simulink library "Simple_lib"  (R2018b)
settings: Solver=ode45  StartTime=0.0  StopTime=10.0  RelTol=1e-3  EnableMultiTasking=on
undefined symbols (not defined in the file or in its folder): Acceptance, beta, C, C_J, C_P, c_wall, dGain, DiscIntNeverNeededParam, Duplex, Electrical_lib, grab, h_fe, i, i3, K_T, Kman, KmanCE, mu_s, n_rev, R_arm, Simplex, systemTs, tau_0, TinIC, Ts, w_0, wallMass, Watch_lib
libraries: $bdroot x407, PlantUtilityBlockset_lib x30, peGeneralControl x22, simulink x11
(part 10 of 14)

== system Simple_lib/Utility/SimplexSav ==
  InPot : Inport
  InFlow : Inport  Tag=NOFLUX  Port=2
  FlowDisplay : Display
  FlowSimplexPlexGraphix2 : Scope
      settings: Tag=Flow
  PotDisplay : Display
  PotSimplexPlexGraphix2 : Scope
      settings: Tag=Pot
  Rate Transition : RateTransition  OutPortSampleTimeMultiple=Ts  OutPortSampleTime=Ts
  OutPot : Outport  Tag=NOFLUX
  tag scope: SimplexSubsystemPlexGraphix2=global
  wires:
  InPot/1 -> Rate Transition/1
  InFlow/1 -> FlowSimplexPlexGraphix2/1, FlowDisplay/1, [SimplexSubsystemPlexGraphix2]
  Rate Transition/1 -> OutPot/1, PotSimplexPlexGraphix2/1, PotDisplay/1

== system Simple_lib/Driveline/Changan Transmission/EMachine ==
  J_eMotor : Subsystem  AncestorBlock=PlantUtilityBlockset_lib/Driveline/InertialState
      mask Display:
      | %color('white');
      | %plot([-1 4],[1 1]);
      | %plot([-1 4],[-1 -1]);
      | %color('black')
      | %plot([1 4],[0 0]);
      | plot([-1 -.9 -.5 0 .5 .9 1  .9  .5  0 -.5 -.9 -1],      [ 0  .5 .9 1 .9 .5 0 -.5 -.9 -1 -.9 -.5  0]);
      | %plot([4 4.5 4.5 4],[0 -0.25 0.25 0])
  Transducer : Subsystem
  V : Outport
  w : Outport  Port=2
  wires:
  J_eMotor/1(Out1) -> w/1, Transducer/1(w)
  Transducer/1(V) -> V/1

== system Simple_lib/Driveline/Changan Transmission/FD1 ==
  In1 : Inport
  Pull : Subsystem  Tag=Electrical  AncestorBlock=PlantUtilityBlockset_lib/Utility/Pull  InitFcn=initDuplex
      mask Display:
      | color('white')
      | plot([0 3], [2 2])
      | plot([0 3], [-2 -2])
      | color('black')
      | 
      | plot([0 1 1], [0 0 0.4])
      | plot([1 1 3], [0.6 1 1])
      | plot([1 3 2 1 0 2], [0.6 0.6 0.4 0.6 0.4 0.4])
      | patch([0 2 1],[0.4 0.4 0.6],[0,0,0])
      | plot([3 2 2], [1 1 0.6])
      | plot([2 2 3], [0.4 -1 -1])
  Push : Subsystem  AncestorBlock=PlantUtilityBlockset_lib/Utility/Push  InitFcn=initSimplex
      mask Display:
      | color('white')
      | plot([0 3], [2 2])
      | plot([0 3], [-2 -2])
      | color('black')
      | 
      | plot([0 2 2 3], [1 1 0 0])
      | plot([1 3 2 1 0 2], [0.6 0.6 0.4 0.6 0.4 0.4])
      | patch([1 3 2],[0.6 0.6 0.4],[0,0,0])
      | plot([0 1 1], [1 1 0.6])
      | plot([1 1 0], [0.4 -1 -1])
  ratio : Gain  Gain=n_i/n_o
  speed ratio : Gain  Gain=n_i/n_o
  Out1 : Outport
  wires:
  Pull/1(OutPot) -> Out1/1
  In1/1 -> Push/1(InPot)
  ratio/1 -> Push/2(InFlow)
  Pull/2(OutFlow) -> ratio/1
  speed ratio/1 -> Pull/1(InPot)
  Push/1(OutPot) -> speed ratio/1

== system Simple_lib/Driveline/Changan Transmission/FD2 ==
  In1 : Inport
  Pull : Subsystem  Tag=Electrical  AncestorBlock=PlantUtilityBlockset_lib/Utility/Pull  InitFcn=initDuplex
      mask Display:
      | color('white')
      | plot([0 3], [2 2])
      | plot([0 3], [-2 -2])
      | color('black')
      | 
      | plot([0 1 1], [0 0 0.4])
      | plot([1 1 3], [0.6 1 1])
      | plot([1 3 2 1 0 2], [0.6 0.6 0.4 0.6 0.4 0.4])
      | patch([0 2 1],[0.4 0.4 0.6],[0,0,0])
      | plot([3 2 2], [1 1 0.6])
      | plot([2 2 3], [0.4 -1 -1])
  Push : Subsystem  AncestorBlock=PlantUtilityBlockset_lib/Utility/Push  InitFcn=initSimplex
      mask Display:
      | color('white')
      | plot([0 3], [2 2])
      | plot([0 3], [-2 -2])
      | color('black')
      | 
      | plot([0 2 2 3], [1 1 0 0])
      | plot([1 3 2 1 0 2], [0.6 0.6 0.4 0.6 0.4 0.4])
      | patch([1 3 2],[0.6 0.6 0.4],[0,0,0])
      | plot([0 1 1], [1 1 0.6])
      | plot([1 1 0], [0.4 -1 -1])
  ratio : Gain  Gain=n_i/n_o
  speed ratio : Gain  Gain=n_i/n_o
  Out1 : Outport
  wires:
  Pull/1(OutPot) -> Out1/1
  In1/1 -> Push/1(InPot)
  ratio/1 -> Push/2(InFlow)
  Pull/2(OutFlow) -> ratio/1
  speed ratio/1 -> Pull/1(InPot)
  Push/1(OutPot) -> speed ratio/1

== system Simple_lib/Driveline/Changan Transmission/GP1 ==
  In1 : Inport
  Pull : Subsystem  Tag=Electrical  AncestorBlock=PlantUtilityBlockset_lib/Utility/Pull  InitFcn=initDuplex
      mask Display:
      | color('white')
      | plot([0 3], [2 2])
      | plot([0 3], [-2 -2])
      | color('black')
      | 
      | plot([0 1 1], [0 0 0.4])
      | plot([1 1 3], [0.6 1 1])
      | plot([1 3 2 1 0 2], [0.6 0.6 0.4 0.6 0.4 0.4])
      | patch([0 2 1],[0.4 0.4 0.6],[0,0,0])
      | plot([3 2 2], [1 1 0.6])
      | plot([2 2 3], [0.4 -1 -1])
  Push : Subsystem  AncestorBlock=PlantUtilityBlockset_lib/Utility/Push  InitFcn=initSimplex
      mask Display:
      | color('white')
      | plot([0 3], [2 2])
      | plot([0 3], [-2 -2])
      | color('black')
      | 
      | plot([0 2 2 3], [1 1 0 0])
      | plot([1 3 2 1 0 2], [0.6 0.6 0.4 0.6 0.4 0.4])
      | patch([1 3 2],[0.6 0.6 0.4],[0,0,0])
      | plot([0 1 1], [1 1 0.6])
      | plot([1 1 0], [0.4 -1 -1])
  ratio : Gain  Gain=n_i/n_o
  speed ratio : Gain  Gain=n_i/n_o
  Out1 : Outport
  wires:
  Pull/1(OutPot) -> Out1/1
  In1/1 -> Push/1(InPot)
  ratio/1 -> Push/2(InFlow)
  Pull/2(OutFlow) -> ratio/1
  speed ratio/1 -> Pull/1(InPot)
  Push/1(OutPot) -> speed ratio/1

== system Simple_lib/Driveline/Changan Transmission/GP2 ==
  In1 : Inport
  Pull : Subsystem  Tag=Electrical  AncestorBlock=PlantUtilityBlockset_lib/Utility/Pull  InitFcn=initDuplex
      mask Display:
      | color('white')
      | plot([0 3], [2 2])
      | plot([0 3], [-2 -2])
      | color('black')
      | 
      | plot([0 1 1], [0 0 0.4])
      | plot([1 1 3], [0.6 1 1])
      | plot([1 3 2 1 0 2], [0.6 0.6 0.4 0.6 0.4 0.4])
      | patch([0 2 1],[0.4 0.4 0.6],[0,0,0])
      | plot([3 2 2], [1 1 0.6])
      | plot([2 2 3], [0.4 -1 -1])
  Push : Subsystem  AncestorBlock=PlantUtilityBlockset_lib/Utility/Push  InitFcn=initSimplex
      mask Display:
      | color('white')
      | plot([0 3], [2 2])
      | plot([0 3], [-2 -2])
      | color('black')
      | 
      | plot([0 2 2 3], [1 1 0 0])
      | plot([1 3 2 1 0 2], [0.6 0.6 0.4 0.6 0.4 0.4])
      | patch([1 3 2],[0.6 0.6 0.4],[0,0,0])
      | plot([0 1 1], [1 1 0.6])
      | plot([1 1 0], [0.4 -1 -1])
  ratio : Gain  Gain=n_i/n_o
  speed ratio : Gain  Gain=n_i/n_o
  Out1 : Outport
  wires:
  Pull/1(OutPot) -> Out1/1
  In1/1 -> Push/1(InPot)
  ratio/1 -> Push/2(InFlow)
  Pull/2(OutFlow) -> ratio/1
  speed ratio/1 -> Pull/1(InPot)
  Push/1(OutPot) -> speed ratio/1

== system Simple_lib/Driveline/Changan Transmission/GP3 ==
  In1 : Inport
  Pull : Subsystem  Tag=Electrical  AncestorBlock=PlantUtilityBlockset_lib/Utility/Pull  InitFcn=initDuplex
      mask Display:
      | color('white')
      | plot([0 3], [2 2])
      | plot([0 3], [-2 -2])
      | color('black')
      | 
      | plot([0 1 1], [0 0 0.4])
      | plot([1 1 3], [0.6 1 1])
      | plot([1 3 2 1 0 2], [0.6 0.6 0.4 0.6 0.4 0.4])
      | patch([0 2 1],[0.4 0.4 0.6],[0,0,0])
      | plot([3 2 2], [1 1 0.6])
      | plot([2 2 3], [0.4 -1 -1])
  Push : Subsystem  AncestorBlock=PlantUtilityBlockset_lib/Utility/Push  InitFcn=initSimplex
      mask Display:
      | color('white')
      | plot([0 3], [2 2])
      | plot([0 3], [-2 -2])
      | color('black')
      | 
      | plot([0 2 2 3], [1 1 0 0])
      | plot([1 3 2 1 0 2], [0.6 0.6 0.4 0.6 0.4 0.4])
      | patch([1 3 2],[0.6 0.6 0.4],[0,0,0])
      | plot([0 1 1], [1 1 0.6])
      | plot([1 1 0], [0.4 -1 -1])
  ratio : Gain  Gain=n_i/n_o
  speed ratio : Gain  Gain=n_i/n_o
  Out1 : Outport
  wires:
  Pull/1(OutPot) -> Out1/1
  In1/1 -> Push/1(InPot)
  ratio/1 -> Push/2(InFlow)
  Pull/2(OutFlow) -> ratio/1
  speed ratio/1 -> Pull/1(InPot)
  Push/1(OutPot) -> speed ratio/1

== system Simple_lib/Driveline/Changan Transmission/GP4  ==
  In1 : Inport
  Pull : Subsystem  Tag=Electrical  AncestorBlock=PlantUtilityBlockset_lib/Utility/Pull  InitFcn=initDuplex
      mask Display:
      | color('white')
      | plot([0 3], [2 2])
      | plot([0 3], [-2 -2])
      | color('black')
      | 
      | plot([0 1 1], [0 0 0.4])
      | plot([1 1 3], [0.6 1 1])
      | plot([1 3 2 1 0 2], [0.6 0.6 0.4 0.6 0.4 0.4])
      | patch([0 2 1],[0.4 0.4 0.6],[0,0,0])
      | plot([3 2 2], [1 1 0.6])
      | plot([2 2 3], [0.4 -1 -1])
  Push : Subsystem  AncestorBlock=PlantUtilityBlockset_lib/Utility/Push  InitFcn=initSimplex
      mask Display:
      | color('white')
      | plot([0 3], [2 2])
      | plot([0 3], [-2 -2])
      | color('black')
      | 
      | plot([0 2 2 3], [1 1 0 0])
      | plot([1 3 2 1 0 2], [0.6 0.6 0.4 0.6 0.4 0.4])
      | patch([1 3 2],[0.6 0.6 0.4],[0,0,0])
      | plot([0 1 1], [1 1 0.6])
      | plot([1 1 0], [0.4 -1 -1])
  ratio : Gain  Gain=n_i/n_o
  speed ratio : Gain  Gain=n_i/n_o
  Out1 : Outport
  wires:
  Pull/1(OutPot) -> Out1/1
  In1/1 -> Push/1(InPot)
  ratio/1 -> Push/2(InFlow)
  Pull/2(OutFlow) -> ratio/1
  speed ratio/1 -> Pull/1(InPot)
  Push/1(OutPot) -> speed ratio/1

== system Simple_lib/Driveline/Changan Transmission/GP5 ==
  In1 : Inport
  Pull : Subsystem  Tag=Electrical  AncestorBlock=PlantUtilityBlockset_lib/Utility/Pull  InitFcn=initDuplex
      mask Display:
      | color('white')
      | plot([0 3], [2 2])
      | plot([0 3], [-2 -2])
      | color('black')
      | 
      | plot([0 1 1], [0 0 0.4])
      | plot([1 1 3], [0.6 1 1])
      | plot([1 3 2 1 0 2], [0.6 0.6 0.4 0.6 0.4 0.4])
      | patch([0 2 1],[0.4 0.4 0.6],[0,0,0])
      | plot([3 2 2], [1 1 0.6])
      | plot([2 2 3], [0.4 -1 -1])
  Push : Subsystem  AncestorBlock=PlantUtilityBlockset_lib/Utility/Push  InitFcn=initSimplex
      mask Display:
      | color('white')
      | plot([0 3], [2 2])
      | plot([0 3], [-2 -2])
      | color('black')
      | 
      | plot([0 2 2 3], [1 1 0 0])
      | plot([1 3 2 1 0 2], [0.6 0.6 0.4 0.6 0.4 0.4])
      | patch([1 3 2],[0.6 0.6 0.4],[0,0,0])
      | plot([0 1 1], [1 1 0.6])
      | plot([1 1 0], [0.4 -1 -1])
  ratio : Gain  Gain=n_i/n_o
  speed ratio : Gain  Gain=n_i/n_o
  Out1 : Outport
  wires:
  Pull/1(OutPot) -> Out1/1
  In1/1 -> Push/1(InPot)
  ratio/1 -> Push/2(InFlow)
  Pull/2(OutFlow) -> ratio/1
  speed ratio/1 -> Pull/1(InPot)
  Push/1(OutPot) -> speed ratio/1

== system Simple_lib/Driveline/Changan Transmission/GP6 ==
  In1 : Inport
  Pull : Subsystem  Tag=Electrical  AncestorBlock=PlantUtilityBlockset_lib/Utility/Pull  InitFcn=initDuplex
      mask Display:
      | color('white')
      | plot([0 3], [2 2])
      | plot([0 3], [-2 -2])
      | color('black')
      | 
      | plot([0 1 1], [0 0 0.4])
      | plot([1 1 3], [0.6 1 1])
      | plot([1 3 2 1 0 2], [0.6 0.6 0.4 0.6 0.4 0.4])
      | patch([0 2 1],[0.4 0.4 0.6],[0,0,0])
      | plot([3 2 2], [1 1 0.6])
      | plot([2 2 3], [0.4 -1 -1])
  Push : Subsystem  AncestorBlock=PlantUtilityBlockset_lib/Utility/Push  InitFcn=initSimplex
      mask Display:
      | color('white')
      | plot([0 3], [2 2])
      | plot([0 3], [-2 -2])
      | color('black')
      | 
      | plot([0 2 2 3], [1 1 0 0])
      | plot([1 3 2 1 0 2], [0.6 0.6 0.4 0.6 0.4 0.4])
      | patch([1 3 2],[0.6 0.6 0.4],[0,0,0])
      | plot([0 1 1], [1 1 0.6])
      | plot([1 1 0], [0.4 -1 -1])
  ratio : Gain  Gain=n_i/n_o
  speed ratio : Gain  Gain=n_i/n_o
  Out1 : Outport
  wires:
  Pull/1(OutPot) -> Out1/1
  In1/1 -> Push/1(InPot)
  ratio/1 -> Push/2(InFlow)
  Pull/2(OutFlow) -> ratio/1
  speed ratio/1 -> Pull/1(InPot)
  Push/1(OutPot) -> speed ratio/1

== system Simple_lib/Driveline/Changan Transmission/GPR ==
  In1 : Inport
  Pull : Subsystem  Tag=Electrical  AncestorBlock=PlantUtilityBlockset_lib/Utility/Pull  InitFcn=initDuplex
      mask Display:
      | color('white')
      | plot([0 3], [2 2])
      | plot([0 3], [-2 -2])
      | color('black')
      | 
      | plot([0 1 1], [0 0 0.4])
      | plot([1 1 3], [0.6 1 1])
      | plot([1 3 2 1 0 2], [0.6 0.6 0.4 0.6 0.4 0.4])
      | patch([0 2 1],[0.4 0.4 0.6],[0,0,0])
      | plot([3 2 2], [1 1 0.6])
      | plot([2 2 3], [0.4 -1 -1])
  Push : Subsystem  AncestorBlock=PlantUtilityBlockset_lib/Utility/Push  InitFcn=initSimplex
      mask Display:
      | color('white')
      | plot([0 3], [2 2])
      | plot([0 3], [-2 -2])
      | color('black')
      | 
      | plot([0 2 2 3], [1 1 0 0])
      | plot([1 3 2 1 0 2], [0.6 0.6 0.4 0.6 0.4 0.4])
      | patch([1 3 2],[0.6 0.6 0.4],[0,0,0])
      | plot([0 1 1], [1 1 0.6])
      | plot([1 1 0], [0.4 -1 -1])
  ratio : Gain  Gain=n_i/n_o
  speed ratio : Gain  Gain=n_i/n_o
  Out1 : Outport
  wires:
  Pull/1(OutPot) -> Out1/1
  In1/1 -> Push/1(InPot)
  ratio/1 -> Push/2(InFlow)
  Pull/2(OutFlow) -> ratio/1
  speed ratio/1 -> Pull/1(InPot)
  Push/1(OutPot) -> speed ratio/1

== system Simple_lib/Driveline/Changan Transmission/K0 ==
  w_in : Inport
  cap : Inport  Port=2
  w_out : Inport  Port=3
  1/R1 : Gain  Gain=-1
  1/R4 : Gain  Gain=-1
  Delay : Delay  DelayLength=1  InitialCondition=0
  Dw : Scope
  Dynamic Friction : Subsystem
  Push_in : Subsystem  AncestorBlock=PlantUtilityBlockset_lib/Utility/Push  InitFcn=initSimplex
      mask Display:
      | color('white')
      | plot([0 3], [2 2])
      | plot([0 3], [-2 -2])
      | color('black')
      | 
      | plot([0 2 2 3], [1 1 0 0])
      | plot([1 3 2 1 0 2], [0.6 0.6 0.4 0.6 0.4 0.4])
      | patch([1 3 2],[0.6 0.6 0.4],[0,0,0])
      | plot([0 1 1], [1 1 0.6])
      | plot([1 1 0], [0.4 -1 -1])
  Push_out : Subsystem  AncestorBlock=PlantUtilityBlockset_lib/Utility/Push  InitFcn=initSimplex
      mask Display:
      | color('white')
      | plot([0 3], [2 2])
      | plot([0 3], [-2 -2])
      | color('black')
      | 
      | plot([0 2 2 3], [1 1 0 0])
      | plot([1 3 2 1 0 2], [0.6 0.6 0.4 0.6 0.4 0.4])
      | patch([1 3 2],[0.6 0.6 0.4],[0,0,0])
      | plot([0 1 1], [1 1 0.6])
      | plot([1 1 0], [0.4 -1 -1])
  Static Friction : Subsystem
  Sum : Sum  Inputs=+|+
  Sum1 : Sum  Inputs=+|+
  Tq_Dyn : Scope
  Tq_stat : Scope
  Tq_trans : Scope
  capacity : Scope
  wires:
  w_out/1 -> Push_out/1(InPot)
  w_in/1 -> Push_in/1(InPot)
  1/R4/1 -> Sum/1
  Sum1/1 -> 1/R1/1, Delay/1, Push_in/2(InFlow)
  Sum/1 -> Dynamic Friction/1(Dw), Dw/1, Static Friction/2(Dw)
  Push_out/1(OutPot) -> Static Friction/3(w), Sum/2
  Push_in/1(OutPot) -> 1/R4/1
  Dynamic Friction/1(Tq_dyn) -> Tq_Dyn/1, Sum1/1
  Static Friction/1(Tq_stat) -> Tq_stat/1, Sum1/2
  Delay/1 -> Tq_trans/1, Static Friction/4(Tq)
  cap/1 -> capacity/1, Dynamic Friction/2(cap), Static Friction/1(cap)
  1/R1/1 -> Push_out/2(InFlow)

== system Simple_lib/Driveline/Changan Transmission/K1 ==
  w_in : Inport
  cap : Inport  Port=2
  w_out : Inport  Port=3
  1/R1 : Gain  Gain=-1
  1/R4 : Gain  Gain=-1
  Delay : Delay  DelayLength=1  InitialCondition=0
  Dw : Scope
  Dynamic Friction : Subsystem
  Push_in : Subsystem  AncestorBlock=PlantUtilityBlockset_lib/Utility/Push  InitFcn=initSimplex
      mask Display:
      | color('white')
      | plot([0 3], [2 2])
      | plot([0 3], [-2 -2])
      | color('black')
      | 
      | plot([0 2 2 3], [1 1 0 0])
      | plot([1 3 2 1 0 2], [0.6 0.6 0.4 0.6 0.4 0.4])
      | patch([1 3 2],[0.6 0.6 0.4],[0,0,0])
      | plot([0 1 1], [1 1 0.6])
      | plot([1 1 0], [0.4 -1 -1])
  Push_out : Subsystem  AncestorBlock=PlantUtilityBlockset_lib/Utility/Push  InitFcn=initSimplex
      mask Display:
      | color('white')
      | plot([0 3], [2 2])
      | plot([0 3], [-2 -2])
      | color('black')
      | 
      | plot([0 2 2 3], [1 1 0 0])
      | plot([1 3 2 1 0 2], [0.6 0.6 0.4 0.6 0.4 0.4])
      | patch([1 3 2],[0.6 0.6 0.4],[0,0,0])
      | plot([0 1 1], [1 1 0.6])
      | plot([1 1 0], [0.4 -1 -1])
  Static Friction : Subsystem
  Sum : Sum  Inputs=+|+
  Sum1 : Sum  Inputs=+|+
  Tq_Dyn : Scope
  Tq_stat : Scope
  Tq_trans : Scope
  capacity : Scope
  wires:
  w_out/1 -> Push_out/1(InPot)
  w_in/1 -> Push_in/1(InPot)
  1/R4/1 -> Sum/1
  Sum1/1 -> 1/R1/1, Delay/1, Push_in/2(InFlow)
  Sum/1 -> Dynamic Friction/1(Dw), Dw/1, Static Friction/2(Dw)
  Push_out/1(OutPot) -> Static Friction/3(w), Sum/2
  Push_in/1(OutPot) -> 1/R4/1
  Dynamic Friction/1(Tq_dyn) -> Tq_Dyn/1, Sum1/1
  Static Friction/1(Tq_stat) -> Tq_stat/1, Sum1/2
  Delay/1 -> Tq_trans/1, Static Friction/4(Tq)
  cap/1 -> capacity/1, Dynamic Friction/2(cap), Static Friction/1(cap)
  1/R1/1 -> Push_out/2(InFlow)

== system Simple_lib/Driveline/Changan Transmission/K2 ==
  w_in : Inport
  cap : Inport  Port=2
  w_out : Inport  Port=3
  1/R1 : Gain  Gain=-1
  1/R4 : Gain  Gain=-1
  Delay : Delay  DelayLength=1  InitialCondition=0
  Dw : Scope
  Dynamic Friction : Subsystem
  Push_in : Subsystem  AncestorBlock=PlantUtilityBlockset_lib/Utility/Push  InitFcn=initSimplex
      mask Display:
      | color('white')
      | plot([0 3], [2 2])
      | plot([0 3], [-2 -2])
      | color('black')
      | 
      | plot([0 2 2 3], [1 1 0 0])
      | plot([1 3 2 1 0 2], [0.6 0.6 0.4 0.6 0.4 0.4])
      | patch([1 3 2],[0.6 0.6 0.4],[0,0,0])
      | plot([0 1 1], [1 1 0.6])
      | plot([1 1 0], [0.4 -1 -1])
  Push_out : Subsystem  AncestorBlock=PlantUtilityBlockset_lib/Utility/Push  InitFcn=initSimplex
      mask Display:
      | color('white')
      | plot([0 3], [2 2])
      | plot([0 3], [-2 -2])
      | color('black')
      | 
      | plot([0 2 2 3], [1 1 0 0])
      | plot([1 3 2 1 0 2], [0.6 0.6 0.4 0.6 0.4 0.4])
      | patch([1 3 2],[0.6 0.6 0.4],[0,0,0])
      | plot([0 1 1], [1 1 0.6])
      | plot([1 1 0], [0.4 -1 -1])
  Static Friction : Subsystem
  Sum : Sum  Inputs=+|+
  Sum1 : Sum  Inputs=+|+
  Tq_Dyn : Scope
  Tq_stat : Scope
  Tq_trans : Scope
  capacity : Scope
  wires:
  w_out/1 -> Push_out/1(InPot)
  w_in/1 -> Push_in/1(InPot)
  1/R4/1 -> Sum/1
  Sum1/1 -> 1/R1/1, Delay/1, Push_in/2(InFlow)
  Sum/1 -> Dynamic Friction/1(Dw), Dw/1, Static Friction/2(Dw)
  Push_out/1(OutPot) -> Static Friction/3(w), Sum/2
  Push_in/1(OutPot) -> 1/R4/1
  Dynamic Friction/1(Tq_dyn) -> Tq_Dyn/1, Sum1/1
  Static Friction/1(Tq_stat) -> Tq_stat/1, Sum1/2
  Delay/1 -> Tq_trans/1, Static Friction/4(Tq)
  cap/1 -> capacity/1, Dynamic Friction/2(cap), Static Friction/1(cap)
  1/R1/1 -> Push_out/2(InFlow)

== system Simple_lib/Driveline/Changan Transmission/LoadScopes ==
  In1 : Inport
  Pull : Subsystem  Tag=Electrical  AncestorBlock=PlantUtilityBlockset_lib/Utility/Pull  InitFcn=initDuplex
      mask Display:
      | color('white')
      | plot([0 3], [2 2])
      | plot([0 3], [-2 -2])
      | color('black')
      | 
      | plot([0 1 1], [0 0 0.4])
      | plot([1 1 3], [0.6 1 1])
      | plot([1 3 2 1 0 2], [0.6 0.6 0.4 0.6 0.4 0.4])
      | patch([0 2 1],[0.4 0.4 0.6],[0,0,0])
      | plot([3 2 2], [1 1 0.6])
      | plot([2 2 3], [0.4 -1 -1])
  Push : Subsystem  AncestorBlock=PlantUtilityBlockset_lib/Utility/Push  InitFcn=initSimplex
      mask Display:
      | color('white')
      | plot([0 3], [2 2])
      | plot([0 3], [-2 -2])
      | color('black')
      | 
      | plot([0 2 2 3], [1 1 0 0])
      | plot([1 3 2 1 0 2], [0.6 0.6 0.4 0.6 0.4 0.4])
      | patch([1 3 2],[0.6 0.6 0.4],[0,0,0])
      | plot([0 1 1], [1 1 0.6])
      | plot([1 1 0], [0.4 -1 -1])
  Scope : Scope  NumInputPorts=2
  Out1 : Outport
  wires:
  Pull/1(OutPot) -> Out1/1
  In1/1 -> Push/1(InPot)
  Pull/2(OutFlow) -> Push/2(InFlow), Scope/2
  Push/1(OutPot) -> Scope/1, Pull/1(InPot)

== system Simple_lib/Driveline/Changan Transmission/Requirements ==
  note: Require synchroniser clutches to lock up when speeds across them are small for a while.
  note: Require clutches to lock up when speeds across them are small for a while.
  note: Require correct ratios when in each gear.
  In1 : Inport
  Out1 : Outport
  wires:
  In1/1 -> Out1/1

== system Simple_lib/Driveline/Changan Transmission/Shaft1 ==
  Discrete-Time Integrator1 : DiscreteIntegrator  gainval=1/5  SampleTime=Ts  ICPrevOutput=DiscIntNeverNeededParam  ICPrevScaledInput=DiscIntNeverNeededParam
  Pull : Subsystem  Tag=Electrical  AncestorBlock=PlantUtilityBlockset_lib/Utility/Pull  InitFcn=initDuplex
      mask Display:
      | color('white')
      | plot([0 3], [2 2])
      | plot([0 3], [-2 -2])
      | color('black')
      | 
      | plot([0 1 1], [0 0 0.4])
      | plot([1 1 3], [0.6 1 1])
      | plot([1 3 2 1 0 2], [0.6 0.6 0.4 0.6 0.4 0.4])
      | patch([0 2 1],[0.4 0.4 0.6],[0,0,0])
      | plot([3 2 2], [1 1 0.6])
      | plot([2 2 3], [0.4 -1 -1])
  Out1 : Outport
  wires:
  Discrete-Time Integrator1/1 -> Pull/1(InPot)
  Pull/2(OutFlow) -> Discrete-Time Integrator1/1
  Pull/1(OutPot) -> Out1/1

== system Simple_lib/Driveline/Changan Transmission/Shaft2 ==
  Discrete-Time Integrator1 : DiscreteIntegrator  gainval=1/5  SampleTime=Ts  ICPrevOutput=DiscIntNeverNeededParam  ICPrevScaledInput=DiscIntNeverNeededParam
  Pull : Subsystem  Tag=Electrical  AncestorBlock=PlantUtilityBlockset_lib/Utility/Pull  InitFcn=initDuplex
      mask Display:
      | color('white')
      | plot([0 3], [2 2])
      | plot([0 3], [-2 -2])
      | color('black')
      | 
      | plot([0 1 1], [0 0 0.4])
      | plot([1 1 3], [0.6 1 1])
      | plot([1 3 2 1 0 2], [0.6 0.6 0.4 0.6 0.4 0.4])
      | patch([0 2 1],[0.4 0.4 0.6],[0,0,0])
      | plot([3 2 2], [1 1 0.6])
      | plot([2 2 3], [0.4 -1 -1])
  Out1 : Outport
  wires:
  Discrete-Time Integrator1/1 -> Pull/1(InPot)
  Pull/2(OutFlow) -> Discrete-Time Integrator1/1
  Pull/1(OutPot) -> Out1/1

== system Simple_lib/Driveline/Changan Transmission/Synchro ==
  w_in : Inport
  cap : Inport  Port=2
  w_out : Inport  Port=3
  1/R1 : Gain  Gain=-1
  1/R4 : Gain  Gain=-1
  Delay : Delay  DelayLength=1  InitialCondition=0
  Dw : Scope
  Dynamic Friction : Subsystem
  Push_in : Subsystem  AncestorBlock=PlantUtilityBlockset_lib/Utility/Push  InitFcn=initSimplex
      mask Display:
      | color('white')
      | plot([0 3], [2 2])
      | plot([0 3], [-2 -2])
      | color('black')
      | 
      | plot([0 2 2 3], [1 1 0 0])
      | plot([1 3 2 1 0 2], [0.6 0.6 0.4 0.6 0.4 0.4])
      | patch([1 3 2],[0.6 0.6 0.4],[0,0,0])
      | plot([0 1 1], [1 1 0.6])
      | plot([1 1 0], [0.4 -1 -1])
  Push_out : Subsystem  AncestorBlock=PlantUtilityBlockset_lib/Utility/Push  InitFcn=initSimplex
      mask Display:
      | color('white')
      | plot([0 3], [2 2])
      | plot([0 3], [-2 -2])
      | color('black')
      | 
      | plot([0 2 2 3], [1 1 0 0])
      | plot([1 3 2 1 0 2], [0.6 0.6 0.4 0.6 0.4 0.4])
      | patch([1 3 2],[0.6 0.6 0.4],[0,0,0])
      | plot([0 1 1], [1 1 0.6])
      | plot([1 1 0], [0.4 -1 -1])
  Static Friction : Subsystem
  Sum : Sum  Inputs=+|+
  Sum1 : Sum  Inputs=+|+
  Tq_Dyn : Scope
  Tq_stat : Scope
  Tq_trans : Scope
  capacity : Scope
  wires:
  w_out/1 -> Push_out/1(InPot)
  w_in/1 -> Push_in/1(InPot)
  1/R4/1 -> Sum/1
  Sum1/1 -> 1/R1/1, Delay/1, Push_in/2(InFlow)
  Sum/1 -> Dynamic Friction/1(Dw), Dw/1, Static Friction/2(Dw)
  Push_out/1(OutPot) -> Static Friction/3(w), Sum/2
  Push_in/1(OutPot) -> 1/R4/1
  Dynamic Friction/1(Tq_dyn) -> Tq_Dyn/1, Sum1/1
  Static Friction/1(Tq_stat) -> Tq_stat/1, Sum1/2
  Delay/1 -> Tq_trans/1, Static Friction/4(Tq)
  cap/1 -> capacity/1, Dynamic Friction/2(cap), Static Friction/1(cap)
  1/R1/1 -> Push_out/2(InFlow)

== system Simple_lib/Driveline/Changan Transmission/Synchro1 ==
  w_in : Inport
  cap : Inport  Port=2
  w_out : Inport  Port=3
  1/R1 : Gain  Gain=-1
  1/R4 : Gain  Gain=-1
  Delay : Delay  DelayLength=1  InitialCondition=0
  Dw : Scope
  Dynamic Friction : Subsystem
  Push_in : Subsystem  AncestorBlock=PlantUtilityBlockset_lib/Utility/Push  InitFcn=initSimplex
      mask Display:
      | color('white')
      | plot([0 3], [2 2])
      | plot([0 3], [-2 -2])
      | color('black')
      | 
      | plot([0 2 2 3], [1 1 0 0])
      | plot([1 3 2 1 0 2], [0.6 0.6 0.4 0.6 0.4 0.4])
      | patch([1 3 2],[0.6 0.6 0.4],[0,0,0])
      | plot([0 1 1], [1 1 0.6])
      | plot([1 1 0], [0.4 -1 -1])
  Push_out : Subsystem  AncestorBlock=PlantUtilityBlockset_lib/Utility/Push  InitFcn=initSimplex
      mask Display:
      | color('white')
      | plot([0 3], [2 2])
      | plot([0 3], [-2 -2])
      | color('black')
      | 
      | plot([0 2 2 3], [1 1 0 0])
      | plot([1 3 2 1 0 2], [0.6 0.6 0.4 0.6 0.4 0.4])
      | patch([1 3 2],[0.6 0.6 0.4],[0,0,0])
      | plot([0 1 1], [1 1 0.6])
      | plot([1 1 0], [0.4 -1 -1])
  Static Friction : Subsystem
  Sum : Sum  Inputs=+|+
  Sum1 : Sum  Inputs=+|+
  Tq_Dyn : Scope
  Tq_stat : Scope
  Tq_trans : Scope
  capacity : Scope
  wires:
  w_out/1 -> Push_out/1(InPot)
  w_in/1 -> Push_in/1(InPot)
  1/R4/1 -> Sum/1
  Sum1/1 -> 1/R1/1, Delay/1, Push_in/2(InFlow)
  Sum/1 -> Dynamic Friction/1(Dw), Dw/1, Static Friction/2(Dw)
  Push_out/1(OutPot) -> Static Friction/3(w), Sum/2
  Push_in/1(OutPot) -> 1/R4/1
  Dynamic Friction/1(Tq_dyn) -> Tq_Dyn/1, Sum1/1
  Static Friction/1(Tq_stat) -> Tq_stat/1, Sum1/2
  Delay/1 -> Tq_trans/1, Static Friction/4(Tq)
  cap/1 -> capacity/1, Dynamic Friction/2(cap), Static Friction/1(cap)
  1/R1/1 -> Push_out/2(InFlow)

== system Simple_lib/Driveline/Changan Transmission/Synchro2 ==
  w_in : Inport
  cap : Inport  Port=2
  w_out : Inport  Port=3
  1/R1 : Gain  Gain=-1
  1/R4 : Gain  Gain=-1
  Delay : Delay  DelayLength=1  InitialCondition=0
  Dw : Scope
  Dynamic Friction : Subsystem
  Push_in : Subsystem  AncestorBlock=PlantUtilityBlockset_lib/Utility/Push  InitFcn=initSimplex
      mask Display:
      | color('white')
      | plot([0 3], [2 2])
      | plot([0 3], [-2 -2])
      | color('black')
      | 
      | plot([0 2 2 3], [1 1 0 0])
      | plot([1 3 2 1 0 2], [0.6 0.6 0.4 0.6 0.4 0.4])
      | patch([1 3 2],[0.6 0.6 0.4],[0,0,0])
      | plot([0 1 1], [1 1 0.6])
      | plot([1 1 0], [0.4 -1 -1])
  Push_out : Subsystem  AncestorBlock=PlantUtilityBlockset_lib/Utility/Push  InitFcn=initSimplex
      mask Display:
      | color('white')
      | plot([0 3], [2 2])
      | plot([0 3], [-2 -2])
      | color('black')
      | 
      | plot([0 2 2 3], [1 1 0 0])
      | plot([1 3 2 1 0 2], [0.6 0.6 0.4 0.6 0.4 0.4])
      | patch([1 3 2],[0.6 0.6 0.4],[0,0,0])
      | plot([0 1 1], [1 1 0.6])
      | plot([1 1 0], [0.4 -1 -1])
  Static Friction : Subsystem
  Sum : Sum  Inputs=+|+
  Sum1 : Sum  Inputs=+|+
  Tq_Dyn : Scope
  Tq_stat : Scope
  Tq_trans : Scope
  capacity : Scope
  wires:
  w_out/1 -> Push_out/1(InPot)
  w_in/1 -> Push_in/1(InPot)
  1/R4/1 -> Sum/1
  Sum1/1 -> 1/R1/1, Delay/1, Push_in/2(InFlow)
  Sum/1 -> Dynamic Friction/1(Dw), Dw/1, Static Friction/2(Dw)
  Push_out/1(OutPot) -> Static Friction/3(w), Sum/2
  Push_in/1(OutPot) -> 1/R4/1
  Dynamic Friction/1(Tq_dyn) -> Tq_Dyn/1, Sum1/1
  Static Friction/1(Tq_stat) -> Tq_stat/1, Sum1/2
  Delay/1 -> Tq_trans/1, Static Friction/4(Tq)
  cap/1 -> capacity/1, Dynamic Friction/2(cap), Static Friction/1(cap)
  1/R1/1 -> Push_out/2(InFlow)

== system Simple_lib/Driveline/Changan Transmission/Synchro3 ==
  w_in : Inport
  cap : Inport  Port=2
  w_out : Inport  Port=3
  1/R1 : Gain  Gain=-1
  1/R4 : Gain  Gain=-1
  Delay : Delay  DelayLength=1  InitialCondition=0
  Dw : Scope
  Dynamic Friction : Subsystem
  Push_in : Subsystem  AncestorBlock=PlantUtilityBlockset_lib/Utility/Push  InitFcn=initSimplex
      mask Display:
      | color('white')
      | plot([0 3], [2 2])
      | plot([0 3], [-2 -2])
      | color('black')
      | 
      | plot([0 2 2 3], [1 1 0 0])
      | plot([1 3 2 1 0 2], [0.6 0.6 0.4 0.6 0.4 0.4])
      | patch([1 3 2],[0.6 0.6 0.4],[0,0,0])
      | plot([0 1 1], [1 1 0.6])
      | plot([1 1 0], [0.4 -1 -1])
  Push_out : Subsystem  AncestorBlock=PlantUtilityBlockset_lib/Utility/Push  InitFcn=initSimplex
      mask Display:
      | color('white')
      | plot([0 3], [2 2])
      | plot([0 3], [-2 -2])
      | color('black')
      | 
      | plot([0 2 2 3], [1 1 0 0])
      | plot([1 3 2 1 0 2], [0.6 0.6 0.4 0.6 0.4 0.4])
      | patch([1 3 2],[0.6 0.6 0.4],[0,0,0])
      | plot([0 1 1], [1 1 0.6])
      | plot([1 1 0], [0.4 -1 -1])
  Static Friction : Subsystem
  Sum : Sum  Inputs=+|+
  Sum1 : Sum  Inputs=+|+
  Tq_Dyn : Scope
  Tq_stat : Scope
  Tq_trans : Scope
  capacity : Scope
  wires:
  w_out/1 -> Push_out/1(InPot)
  w_in/1 -> Push_in/1(InPot)
  1/R4/1 -> Sum/1
  Sum1/1 -> 1/R1/1, Delay/1, Push_in/2(InFlow)
  Sum/1 -> Dynamic Friction/1(Dw), Dw/1, Static Friction/2(Dw)
  Push_out/1(OutPot) -> Static Friction/3(w), Sum/2
  Push_in/1(OutPot) -> 1/R4/1
  Dynamic Friction/1(Tq_dyn) -> Tq_Dyn/1, Sum1/1
  Static Friction/1(Tq_stat) -> Tq_stat/1, Sum1/2
  Delay/1 -> Tq_trans/1, Static Friction/4(Tq)
  cap/1 -> capacity/1, Dynamic Friction/2(cap), Static Friction/1(cap)
  1/R1/1 -> Push_out/2(InFlow)

== system Simple_lib/Driveline/Changan Transmission/Synchro4 ==
  w_in : Inport
  cap : Inport  Port=2
  w_out : Inport  Port=3
  1/R1 : Gain  Gain=-1
  1/R4 : Gain  Gain=-1
  Delay : Delay  DelayLength=1  InitialCondition=0
  Dw : Scope
  Dynamic Friction : Subsystem
  Push_in : Subsystem  AncestorBlock=PlantUtilityBlockset_lib/Utility/Push  InitFcn=initSimplex
      mask Display:
      | color('white')
      | plot([0 3], [2 2])
      | plot([0 3], [-2 -2])
      | color('black')
      | 
      | plot([0 2 2 3], [1 1 0 0])
      | plot([1 3 2 1 0 2], [0.6 0.6 0.4 0.6 0.4 0.4])
      | patch([1 3 2],[0.6 0.6 0.4],[0,0,0])
      | plot([0 1 1], [1 1 0.6])
      | plot([1 1 0], [0.4 -1 -1])
  Push_out : Subsystem  AncestorBlock=PlantUtilityBlockset_lib/Utility/Push  InitFcn=initSimplex
      mask Display:
      | color('white')
      | plot([0 3], [2 2])
      | plot([0 3], [-2 -2])
      | color('black')
      | 
      | plot([0 2 2 3], [1 1 0 0])
      | plot([1 3 2 1 0 2], [0.6 0.6 0.4 0.6 0.4 0.4])
      | patch([1 3 2],[0.6 0.6 0.4],[0,0,0])
      | plot([0 1 1], [1 1 0.6])
      | plot([1 1 0], [0.4 -1 -1])
  Static Friction : Subsystem
  Sum : Sum  Inputs=+|+
  Sum1 : Sum  Inputs=+|+
  Tq_Dyn : Scope
  Tq_stat : Scope
  Tq_trans : Scope
  capacity : Scope
  wires:
  w_out/1 -> Push_out/1(InPot)
  w_in/1 -> Push_in/1(InPot)
  1/R4/1 -> Sum/1
  Sum1/1 -> 1/R1/1, Delay/1, Push_in/2(InFlow)
  Sum/1 -> Dynamic Friction/1(Dw), Dw/1, Static Friction/2(Dw)
  Push_out/1(OutPot) -> Static Friction/3(w), Sum/2
  Push_in/1(OutPot) -> 1/R4/1
  Dynamic Friction/1(Tq_dyn) -> Tq_Dyn/1, Sum1/1
  Static Friction/1(Tq_stat) -> Tq_stat/1, Sum1/2
  Delay/1 -> Tq_trans/1, Static Friction/4(Tq)
  cap/1 -> capacity/1, Dynamic Friction/2(cap), Static Friction/1(cap)
  1/R1/1 -> Push_out/2(InFlow)

== system Simple_lib/Driveline/Changan Transmission/Synchro5 ==
  w_in : Inport
  cap : Inport  Port=2
  w_out : Inport  Port=3
  1/R1 : Gain  Gain=-1
  1/R4 : Gain  Gain=-1
  Delay : Delay  DelayLength=1  InitialCondition=0
  Dw : Scope
  Dynamic Friction : Subsystem
  Push_in : Subsystem  AncestorBlock=PlantUtilityBlockset_lib/Utility/Push  InitFcn=initSimplex
      mask Display:
      | color('white')
      | plot([0 3], [2 2])
      | plot([0 3], [-2 -2])
      | color('black')
      | 
      | plot([0 2 2 3], [1 1 0 0])
      | plot([1 3 2 1 0 2], [0.6 0.6 0.4 0.6 0.4 0.4])
      | patch([1 3 2],[0.6 0.6 0.4],[0,0,0])
      | plot([0 1 1], [1 1 0.6])
      | plot([1 1 0], [0.4 -1 -1])
  Push_out : Subsystem  AncestorBlock=PlantUtilityBlockset_lib/Utility/Push  InitFcn=initSimplex
      mask Display:
      | color('white')
      | plot([0 3], [2 2])
      | plot([0 3], [-2 -2])
      | color('black')
      | 
      | plot([0 2 2 3], [1 1 0 0])
      | plot([1 3 2 1 0 2], [0.6 0.6 0.4 0.6 0.4 0.4])
      | patch([1 3 2],[0.6 0.6 0.4],[0,0,0])
      | plot([0 1 1], [1 1 0.6])
      | plot([1 1 0], [0.4 -1 -1])
  Static Friction : Subsystem
  Sum : Sum  Inputs=+|+
  Sum1 : Sum  Inputs=+|+
  Tq_Dyn : Scope
  Tq_stat : Scope
  Tq_trans : Scope
  capacity : Scope
  wires:
  w_out/1 -> Push_out/1(InPot)
  w_in/1 -> Push_in/1(InPot)
  1/R4/1 -> Sum/1
  Sum1/1 -> 1/R1/1, Delay/1, Push_in/2(InFlow)
  Sum/1 -> Dynamic Friction/1(Dw), Dw/1, Static Friction/2(Dw)
  Push_out/1(OutPot) -> Static Friction/3(w), Sum/2
  Push_in/1(OutPot) -> 1/R4/1
  Dynamic Friction/1(Tq_dyn) -> Tq_Dyn/1, Sum1/1
  Static Friction/1(Tq_stat) -> Tq_stat/1, Sum1/2
  Delay/1 -> Tq_trans/1, Static Friction/4(Tq)
  cap/1 -> capacity/1, Dynamic Friction/2(cap), Static Friction/1(cap)
  1/R1/1 -> Push_out/2(InFlow)

== system Simple_lib/Driveline/Changan Transmission/Synchro6 ==
  w_in : Inport
  cap : Inport  Port=2
  w_out : Inport  Port=3
  1/R1 : Gain  Gain=-1
  1/R4 : Gain  Gain=-1
  Delay : Delay  DelayLength=1  InitialCondition=0
  Dw : Scope
  Dynamic Friction : Subsystem
  Push_in : Subsystem  AncestorBlock=PlantUtilityBlockset_lib/Utility/Push  InitFcn=initSimplex
      mask Display:
      | color('white')
      | plot([0 3], [2 2])
      | plot([0 3], [-2 -2])
      | color('black')
      | 
      | plot([0 2 2 3], [1 1 0 0])
      | plot([1 3 2 1 0 2], [0.6 0.6 0.4 0.6 0.4 0.4])
      | patch([1 3 2],[0.6 0.6 0.4],[0,0,0])
      | plot([0 1 1], [1 1 0.6])
      | plot([1 1 0], [0.4 -1 -1])
  Push_out : Subsystem  AncestorBlock=PlantUtilityBlockset_lib/Utility/Push  InitFcn=initSimplex
      mask Display:
      | color('white')
      | plot([0 3], [2 2])
      | plot([0 3], [-2 -2])
      | color('black')
      | 
      | plot([0 2 2 3], [1 1 0 0])
      | plot([1 3 2 1 0 2], [0.6 0.6 0.4 0.6 0.4 0.4])
      | patch([1 3 2],[0.6 0.6 0.4],[0,0,0])
      | plot([0 1 1], [1 1 0.6])
      | plot([1 1 0], [0.4 -1 -1])
  Static Friction : Subsystem
  Sum : Sum  Inputs=+|+
  Sum1 : Sum  Inputs=+|+
  Tq_Dyn : Scope
  Tq_stat : Scope
  Tq_trans : Scope
  capacity : Scope
  wires:
  w_out/1 -> Push_out/1(InPot)
  w_in/1 -> Push_in/1(InPot)
  1/R4/1 -> Sum/1
  Sum1/1 -> 1/R1/1, Delay/1, Push_in/2(InFlow)
  Sum/1 -> Dynamic Friction/1(Dw), Dw/1, Static Friction/2(Dw)
  Push_out/1(OutPot) -> Static Friction/3(w), Sum/2
  Push_in/1(OutPot) -> 1/R4/1
  Dynamic Friction/1(Tq_dyn) -> Tq_Dyn/1, Sum1/1
  Static Friction/1(Tq_stat) -> Tq_stat/1, Sum1/2
  Delay/1 -> Tq_trans/1, Static Friction/4(Tq)
  cap/1 -> capacity/1, Dynamic Friction/2(cap), Static Friction/1(cap)
  1/R1/1 -> Push_out/2(InFlow)

== system Simple_lib/Driveline/Inverter_F/DivideSafely_1 ==
  den : Inport
  num : Inport  Port=2
  Ratio : Product  Inputs=*/
  Switch1 : Switch  Criteria=u2 ~= 0
  Switch2 : Switch  Criteria=u2 ~= 0
  dummy denominator : Constant
  zero denominator return : Constant  Value=tau_0
  rat : Outport
  wires:
  num/1 -> Ratio/1
  zero denominator return/1 -> Switch1/3
  Ratio/1 -> Switch1/1
  Switch1/1 -> rat/1
  dummy denominator/1 -> Switch2/3
  den/1 -> Switch1/2, Switch2/1, Switch2/2
  Switch2/1 -> Ratio/2

== system Simple_lib/Driveline/Inverter_F/DivideSafely_2 ==
  num : Inport
  den : Inport  Port=2
  Ratio : Product  Inputs=*/
  Switch1 : Switch  Criteria=u2 ~= 0
  Switch2 : Switch  Criteria=u2 ~= 0
  dummy denominator : Constant
  zero denominator return : Constant  Value=tau_0
  rat : Outport
  wires:
  num/1 -> Ratio/1
  zero denominator return/1 -> Switch1/3
  Ratio/1 -> Switch1/1
  Switch1/1 -> rat/1
  dummy denominator/1 -> Switch2/3
  den/1 -> Switch1/2, Switch2/1, Switch2/2
  Switch2/1 -> Ratio/2

== system Simple_lib/Driveline/Inverter_F/Simplex ==
  InPot : Inport
  InFlow : Inport  Tag=NOFLUX  Port=2
  OutPot : Outport  Tag=NOFLUX
  tag scope: SimplexInverter_FBEVPlantBEV=global
  wires:
  InPot/1 -> OutPot/1  "SimplexInverter_FBEVPlantBEV"
  InFlow/1 -> [SimplexInverter_FBEVPlantBEV]  "out_SimplexInverter_FBEVPlantBEV"

== system Simple_lib/Driveline/Inverter_F/Simplex1 ==
  InPot : Inport
  InFlow : Inport  Tag=NOFLUX  Port=2
  OutPot : Outport  Tag=NOFLUX
  tag scope: Simplex1Inverter_FBEVPlantBEV=global
  wires:
  InPot/1 -> OutPot/1  "Simplex1Inverter_FBEVPlantBEV"
  InFlow/1 -> [Simplex1Inverter_FBEVPlantBEV]  "out_Simplex1Inverter_FBEVPlantBEV"

== system Simple_lib/Driveline/Inverter_R/DivideSafely_1 ==
  den : Inport
  num : Inport  Port=2
  Ratio : Product  Inputs=*/
  Switch1 : Switch  Criteria=u2 ~= 0
  Switch2 : Switch  Criteria=u2 ~= 0
  dummy denominator : Constant
  zero denominator return : Constant  Value=tau_0
  rat : Outport
  wires:
  num/1 -> Ratio/1
  zero denominator return/1 -> Switch1/3
  Ratio/1 -> Switch1/1
  Switch1/1 -> rat/1
  dummy denominator/1 -> Switch2/3
  den/1 -> Switch1/2, Switch2/1, Switch2/2
  Switch2/1 -> Ratio/2

== system Simple_lib/Driveline/Inverter_R/DivideSafely_2 ==
  num : Inport
  den : Inport  Port=2
  Ratio : Product  Inputs=*/
  Switch1 : Switch  Criteria=u2 ~= 0
  Switch2 : Switch  Criteria=u2 ~= 0
  dummy denominator : Constant
  zero denominator return : Constant  Value=tau_0
  rat : Outport
  wires:
  num/1 -> Ratio/1
  zero denominator return/1 -> Switch1/3
  Ratio/1 -> Switch1/1
  Switch1/1 -> rat/1
  dummy denominator/1 -> Switch2/3
  den/1 -> Switch1/2, Switch2/1, Switch2/2
  Switch2/1 -> Ratio/2

== system Simple_lib/Driveline/Inverter_R/Simplex ==
  InPot : Inport
  InFlow : Inport  Tag=NOFLUX  Port=2
  OutPot : Outport  Tag=NOFLUX
  tag scope: SimplexInverter_RBEVPlantBEV=global
  wires:
  InPot/1 -> OutPot/1  "SimplexInverter_RBEVPlantBEV"
  InFlow/1 -> [SimplexInverter_RBEVPlantBEV]  "out_SimplexInverter_RBEVPlantBEV"

== system Simple_lib/Driveline/Inverter_R/Simplex1 ==
  InPot : Inport
  InFlow : Inport  Tag=NOFLUX  Port=2
  OutPot : Outport  Tag=NOFLUX
  tag scope: Simplex1Inverter_RBEVPlantBEV=global
  wires:
  InPot/1 -> OutPot/1  "Simplex1Inverter_RBEVPlantBEV"
  InFlow/1 -> [Simplex1Inverter_RBEVPlantBEV]  "out_Simplex1Inverter_RBEVPlantBEV"

== system Simple_lib/Driveline/Pseudo Locking Clutch/Dynamic Friction ==
  Dw : Inport
  cap : Inport  Port=2
  Product : Product  RndMeth=Zero
  Saturation : Saturate  UpperLimit=inf  LowerLimit=0
  friction : Trigonometry  Operator=tanh
  grab : Gain  Gain=grab
  Tq_dyn : Outport
  wires:
  Product/1 -> Tq_dyn/1
  Saturation/1 -> Product/1
  cap/1 -> Saturation/1
  friction/1 -> Product/2
  grab/1 -> friction/1
  Dw/1 -> grab/1

== system Simple_lib/Driveline/Pseudo Locking Clutch/Push_in ==
  InPot : Inport
  InFlow : Inport  Tag=NOFLUX  Port=2
  OutPot : Outport  Tag=NOFLUX
  tag scope: Push_inClutchPseudoLockingClutch_test=global
  wires:
  InFlow/1 -> [Push_inClutchPseudoLockingClutch_test]  "flow"
  InPot/1 -> OutPot/1  "pot"

== system Simple_lib/Driveline/Pseudo Locking Clutch/Push_out ==
  InPot : Inport
  InFlow : Inport  Tag=NOFLUX  Port=2
  OutPot : Outport  Tag=NOFLUX
  tag scope: Push_outClutchPseudoLockingClutch_test=global
  wires:
  InFlow/1 -> [Push_outClutchPseudoLockingClutch_test]  "flow"
  InPot/1 -> OutPot/1  "pot"

== system Simple_lib/Driveline/Pseudo Locking Clutch/Static Friction ==
  cap : Inport
  Dw : Inport  Port=2
  w : Inport  Port=3
  Tq : Inport  Port=4
  1/R2 : Gain  Gain=mu_s/2
  Abs : Abs
  Abs1 : Abs
  Abs2 : Abs
  Delay : Delay  DelayLength=1  InitialCondition=0
  Discrete-Time Integrator : DiscreteIntegrator  gainval=k_static  ExternalReset=level  SampleTime=Ts  ICPrevOutput=DiscIntNeverNeededParam  ICPrevScaledInput=DiscIntNeverNeededParam
  Logical Operator : Logic  Operator=OR  AllPortsSameDT=off  OutDataTypeStr=boolean
  Logical Operator1 : Logic  AllPortsSameDT=off  OutDataTypeStr=boolean
  Logical Operator2 : Logic  Operator=NOT  Inputs=1  AllPortsSameDT=off  OutDataTypeStr=boolean
  Relational Operator : RelationalOperator  OutDataTypeStr=boolean  RndMeth=Nearest
  Relational Operator1 : RelationalOperator  OutDataTypeStr=boolean  RndMeth=Nearest
  Saturation1 : Saturate  UpperLimit=inf  LowerLimit=0
  Sum2 : Sum  Inputs=-++
  big speed diff : Scope
  capacity : Scope
  oldtrans_exceeds_cap : Scope
  slipping : Scope
  Tq_stat : Outport
  wires:
  Logical Operator2/1 -> Logical Operator1/2
  Delay/1 -> Logical Operator2/1
  Relational Operator1/1 -> Logical Operator1/1, Delay/1
  Dw/1 -> Sum2/1, Abs/1, Discrete-Time Integrator/1
  w/1 -> Sum2/3, Sum2/2
  Tq/1 -> Abs2/1
  Sum2/1 -> Abs1/1
  Logical Operator1/1 -> Logical Operator/2, oldtrans_exceeds_cap/1
  Abs1/1 -> 1/R2/1
  Saturation1/1 -> Relational Operator1/2
  Abs2/1 -> Relational Operator1/1
  Abs/1 -> Relational Operator/1
  Discrete-Time Integrator/1 -> Tq_stat/1
  Logical Operator/1 -> Discrete-Time Integrator/2, slipping/1
  cap/1 -> Saturation1/1, capacity/1
  Relational Operator/1 -> big speed diff/1, Logical Operator/1
  1/R2/1 -> Relational Operator/2

== system Simple_lib/Driveline/Synchro/Dynamic Friction ==
  note: \tau_{dyn} = | \kappa | tanh( \gamma \Delta \omega )
  Dw : Inport
  cap : Inport  Port=2
  Product : Product  RndMeth=Zero
  Saturation : Saturate  UpperLimit=inf  LowerLimit=0
  friction : Trigonometry  Operator=tanh
  grab : Gain  Gain=grab
  Tq_dyn : Outport
  wires:
  Product/1 -> Tq_dyn/1
  Saturation/1 -> Product/2
  cap/1 -> Saturation/1
  friction/1 -> Product/1
  grab/1 -> friction/1
  Dw/1 -> grab/1

== system Simple_lib/Driveline/Synchro/Static Friction ==
  note: \tau_{stat}  =  0        ( |\tau|>\kappa  \cap  |\Delta\omega|<\mu_s|\omega| )
      |             k_{stat} \int \Delta\omega dt    (otherwise)
  cap : Inport
  Dw : Inport  Port=2
  w : Inport  Port=3
  Tq : Inport  Port=4
  1/R2 : Gain  Gain=mu_s/2
  Abs : Abs
  Abs1 : Abs
  Abs2 : Abs
  Delay : Delay  DelayLength=1  InitialCondition=0
  Discrete-Time Integrator : DiscreteIntegrator  gainval=k_static  ExternalReset=level  SampleTime=Ts  ICPrevOutput=DiscIntNeverNeededParam  ICPrevScaledInput=DiscIntNeverNeededParam
  Logical Operator : Logic  Operator=OR  AllPortsSameDT=off  OutDataTypeStr=boolean
  Logical Operator1 : Logic  AllPortsSameDT=off  OutDataTypeStr=boolean
  Logical Operator2 : Logic  Operator=NOT  Inputs=1  AllPortsSameDT=off  OutDataTypeStr=boolean
  Relational Operator : RelationalOperator  OutDataTypeStr=boolean  RndMeth=Nearest
  Relational Operator1 : RelationalOperator  OutDataTypeStr=boolean  RndMeth=Nearest
  Saturation1 : Saturate  UpperLimit=inf  LowerLimit=0
  Sum2 : Sum  Inputs=++-
  Tq_stat : Outport
  wires:
  Logical Operator2/1 -> Logical Operator1/2
  Delay/1 -> Logical Operator2/1
  Relational Operator1/1 -> Delay/1, Logical Operator1/1
  Dw/1 -> Discrete-Time Integrator/1, Sum2/3, Abs/1
  w/1 -> Sum2/1, Sum2/2
  Tq/1 -> Abs2/1
  Sum2/1 -> Abs1/1
  Logical Operator1/1 -> Logical Operator/1
  Abs1/1 -> 1/R2/1
  Saturation1/1 -> Relational Operator1/2
  Abs2/1 -> Relational Operator1/1
  Abs/1 -> Relational Operator/1
  Discrete-Time Integrator/1 -> Tq_stat/1
  Logical Operator/1 -> Discrete-Time Integrator/2
  cap/1 -> Saturation1/1
  Relational Operator/1 -> Logical Operator/2
  1/R2/1 -> Relational Operator/2

== system Simple_lib/Driveline/Synchro1/Dynamic Friction ==
  Dw : Inport
  cap : Inport  Port=2
  Product : Product  RndMeth=Zero
  Saturation : Saturate  UpperLimit=inf  LowerLimit=0
  friction : Trigonometry  Operator=tanh
  grab : Gain  Gain=grab
  Tq_dyn : Outport
  wires:
  Dw/1 -> grab/1
  grab/1 -> friction/1
  friction/1 -> Product/2
  cap/1 -> Saturation/1
  Saturation/1 -> Product/1
  Product/1 -> Tq_dyn/1

== system Simple_lib/Driveline/Synchro1/Static Friction ==
  cap : Inport
  Dw : Inport  Port=2
  w : Inport  Port=3
  Tq : Inport  Port=4
  1/R2 : Gain  Gain=mu_s/2
  Abs : Abs
  Abs1 : Abs
  Abs2 : Abs
  Delay : Delay  DelayLength=1  InitialCondition=0
  Discrete-Time Integrator : DiscreteIntegrator  gainval=k_static  ExternalReset=level  SampleTime=Ts  ICPrevOutput=DiscIntNeverNeededParam  ICPrevScaledInput=DiscIntNeverNeededParam
  Logical Operator : Logic  Operator=OR  AllPortsSameDT=off  OutDataTypeStr=boolean
  Logical Operator1 : Logic  AllPortsSameDT=off  OutDataTypeStr=boolean
  Logical Operator2 : Logic  Operator=NOT  Inputs=1  AllPortsSameDT=off  OutDataTypeStr=boolean
  Relational Operator : RelationalOperator  OutDataTypeStr=boolean  RndMeth=Nearest
  Relational Operator1 : RelationalOperator  OutDataTypeStr=boolean  RndMeth=Nearest
  Saturation1 : Saturate  UpperLimit=inf  LowerLimit=0
  Sum2 : Sum  Inputs=-++
  big speed diff : Scope
  capacity : Scope
  oldtrans_exceeds_cap : Scope
  slipping : Scope
  Tq_stat : Outport
  wires:
  1/R2/1 -> Relational Operator/2
  Relational Operator/1 -> Logical Operator/1, big speed diff/1
  cap/1 -> capacity/1, Saturation1/1
  Logical Operator/1 -> slipping/1, Discrete-Time Integrator/2
  Discrete-Time Integrator/1 -> Tq_stat/1
  Abs/1 -> Relational Operator/1
  Abs2/1 -> Relational Operator1/1
  Saturation1/1 -> Relational Operator1/2
  Abs1/1 -> 1/R2/1
  Logical Operator1/1 -> oldtrans_exceeds_cap/1, Logical Operator/2
  Sum2/1 -> Abs1/1
  Tq/1 -> Abs2/1
  w/1 -> Sum2/2, Sum2/3
  Dw/1 -> Discrete-Time Integrator/1, Abs/1, Sum2/1
  Relational Operator1/1 -> Delay/1, Logical Operator1/1
  Delay/1 -> Logical Operator2/1
  Logical Operator2/1 -> Logical Operator1/2

== system Simple_lib/Driveline/Torque Source/Simplex ==
  InPot : Inport
  InFlow : Inport  Tag=NOFLUX  Port=2
  OutPot : Outport  Tag=NOFLUX
  tag scope: SimplexResistanceTorqueSourceHybpt_test=global
  wires:
  InPot/1 -> OutPot/1
  InFlow/1 -> [SimplexResistanceTorqueSourceHybpt_test]

== system Simple_lib/Driveline/diff_R/Carrier ==
  note: The diff splits the torque equally
      | and returns the mean speed
  w_in_1 : Inport
  w_in_2 : Inport  Port=2
  Duplex : Subsystem  Tag=Electrical  AncestorBlock=PlantUtilityBlockset_lib/Utility/Pull  InitFcn=initDuplex
      mask Display:
      | color('white')
      | plot([0 3], [2 2])
      | plot([0 3], [-2 -2])
      | color('black')
      | 
      | plot([0 1 1], [0 0 0.4])
      | plot([1 1 3], [0.6 1 1])
      | plot([1 3 2 1 0 2], [0.6 0.6 0.4 0.6 0.4 0.4])
      | patch([0 2 1],[0.4 0.4 0.6],[0,0,0])
      | plot([3 2 2], [1 1 0.6])
      | plot([2 2 3], [0.4 -1 -1])
  Gain : Gain  Gain=1/2
  Gain1 : Gain  Gain=1/2
  Simplex : Subsystem  Tag=Electrical  AncestorBlock=PlantUtilityBlockset_lib/Utility/Push  InitFcn=initSimplex
      mask Display:
      | color('white')
      | plot([0 3], [2 2])
      | plot([0 3], [-2 -2])
      | color('black')
      | 
      | plot([0 2 2 3], [1 1 0 0])
      | plot([1 3 2 1 0 2], [0.6 0.6 0.4 0.6 0.4 0.4])
      | patch([1 3 2],[0.6 0.6 0.4],[0,0,0])
      | plot([0 1 1], [1 1 0.6])
      | plot([1 1 0], [0.4 -1 -1])
  Simplex1 : Subsystem  Tag=Electrical  AncestorBlock=PlantUtilityBlockset_lib/Utility/Push  InitFcn=initSimplex
      mask Display:
      | color('white')
      | plot([0 3], [2 2])
      | plot([0 3], [-2 -2])
      | color('black')
      | 
      | plot([0 2 2 3], [1 1 0 0])
      | plot([1 3 2 1 0 2], [0.6 0.6 0.4 0.6 0.4 0.4])
      | patch([1 3 2],[0.6 0.6 0.4],[0,0,0])
      | plot([0 1 1], [1 1 0.6])
      | plot([1 1 0], [0.4 -1 -1])
  Sum1 : Sum  Inputs=|++
  w_out : Outport
  wires:
  Duplex/1(OutPot) -> w_out/1
  Simplex/1(OutPot) -> Sum1/1
  Duplex/2(OutFlow) -> Gain1/1
  Simplex1/1(OutPot) -> Sum1/2
  Sum1/1 -> Gain/1
  w_in_1/1 -> Simplex/1(InPot)
  w_in_2/1 -> Simplex1/1(InPot)
  Gain/1 -> Duplex/1(InPot)
  Gain1/1 -> Simplex1/2(InFlow), Simplex/2(InFlow)

== system Simple_lib/Driveline/diff_R/GearPair  ==
  In1 : Inport
  Pull : Subsystem  Tag=Electrical  AncestorBlock=PlantUtilityBlockset_lib/Utility/Pull  InitFcn=initDuplex
      mask Display:
      | color('white')
      | plot([0 3], [2 2])
      | plot([0 3], [-2 -2])
      | color('black')
      | 
      | plot([0 1 1], [0 0 0.4])
      | plot([1 1 3], [0.6 1 1])
      | plot([1 3 2 1 0 2], [0.6 0.6 0.4 0.6 0.4 0.4])
      | patch([0 2 1],[0.4 0.4 0.6],[0,0,0])
      | plot([3 2 2], [1 1 0.6])
      | plot([2 2 3], [0.4 -1 -1])
  Push : Subsystem  AncestorBlock=PlantUtilityBlockset_lib/Utility/Push  InitFcn=initSimplex
      mask Display:
      | color('white')
      | plot([0 3], [2 2])
      | plot([0 3], [-2 -2])
      | color('black')
      | 
      | plot([0 2 2 3], [1 1 0 0])
      | plot([1 3 2 1 0 2], [0.6 0.6 0.4 0.6 0.4 0.4])
      | patch([1 3 2],[0.6 0.6 0.4],[0,0,0])
      | plot([0 1 1], [1 1 0.6])
      | plot([1 1 0], [0.4 -1 -1])
  ratio : Gain  Gain=n_i/n_o
  speed ratio : Gain  Gain=n_i/n_o
  Out1 : Outport
  wires:
  Pull/1(OutPot) -> Out1/1
  In1/1 -> Push/1(InPot)
  ratio/1 -> Push/2(InFlow)
  Pull/2(OutFlow) -> ratio/1
  speed ratio/1 -> Pull/1(InPot)
  Push/1(OutPot) -> speed ratio/1

== system Simple_lib/Driveline/diff_R/GearPair 1 ==
  In1 : Inport
  Pull : Subsystem  Tag=Electrical  AncestorBlock=PlantUtilityBlockset_lib/Utility/Pull  InitFcn=initDuplex
      mask Display:
      | color('white')
      | plot([0 3], [2 2])
      | plot([0 3], [-2 -2])
      | color('black')
      | 
      | plot([0 1 1], [0 0 0.4])
      | plot([1 1 3], [0.6 1 1])
      | plot([1 3 2 1 0 2], [0.6 0.6 0.4 0.6 0.4 0.4])
      | patch([0 2 1],[0.4 0.4 0.6],[0,0,0])
      | plot([3 2 2], [1 1 0.6])
      | plot([2 2 3], [0.4 -1 -1])
  Push : Subsystem  AncestorBlock=PlantUtilityBlockset_lib/Utility/Push  InitFcn=initSimplex
      mask Display:
      | color('white')
      | plot([0 3], [2 2])
      | plot([0 3], [-2 -2])
      | color('black')
      | 
      | plot([0 2 2 3], [1 1 0 0])
      | plot([1 3 2 1 0 2], [0.6 0.6 0.4 0.6 0.4 0.4])
      | patch([1 3 2],[0.6 0.6 0.4],[0,0,0])
      | plot([0 1 1], [1 1 0.6])
      | plot([1 1 0], [0.4 -1 -1])
  ratio : Gain  Gain=n_i/n_o
  speed ratio : Gain  Gain=n_i/n_o
  Out1 : Outport
  wires:
  Pull/1(OutPot) -> Out1/1
  In1/1 -> Push/1(InPot)
  ratio/1 -> Push/2(InFlow)
  Pull/2(OutFlow) -> ratio/1
  speed ratio/1 -> Pull/1(InPot)
  Push/1(OutPot) -> speed ratio/1
